simulink model "Linearization2"  (R2022a)
settings: Solver=VariableStepAuto  StartTime=0.0  StopTime=10.0  RelTol=1e-3
undefined symbols (not defined in the file): Aactuator, ac, AeroCoeff, ControlAllocation, DUmax, DUmin, EngineTable, F, fcs, ft, g, hground, IC, kg, LandingGear, Light, LPmethod, m, MIL, Mode_deflection_aileron, Mode_deflection_elevator, Mode_deflection_rudder, Mode_deflection_TVC_y, Mode_deflection_TVC_z, N, Ninv_2nozzle, Ninv_no_nozzle, PIController, s, Sensor, slug, state0, sysID_DAQ, sysID_OBES, Umax_2nozzle, Umax_no_nozzle, Umin_2nozzle, Umin_no_nozzle, WMM2020
libraries: aerolibconvert2 x19, slpidlib x6, simulink x6, sharedutil x4, aerolibatmos2 x3, aerolibwind2 x3, aerolibbdyn x3, aerolibgravity2 x2, sharedtransform x1
(part 4 of 9)

== system Linearization2/F-16 Vehicle Systems Model/sysID_Onboard_Excitation_System/signal generator8 ==
  note: ROM記憶體的指標(Pointer)
  note: 唯讀記憶體，裡面存放波形
  isTurnOn : Inport
  Enable : Inport  Port=2
  sysID_isDone : Inport  Port=3
  Constant1 : Constant  Value=sysID_OBES.rudder.amplitude
  Index Vector : MultiPortSwitch  Inputs=1  SaturateOnIntegerOverflow=off  InputSameDT=off
  Logical Operator1 : Logic  AllPortsSameDT=off  OutDataTypeStr=boolean
  Logical Operator3 : Logic  Operator=NOT  AllPortsSameDT=off  OutDataTypeStr=boolean
  Logical Operator4 : Logic  AllPortsSameDT=off  OutDataTypeStr=boolean
  Pause Counter : Subsystem  TreatAsAtomicUnit=on
  Product : Product
  ROM : Constant  Value=sysID_OBES.rudder.wave
  rudder_delay : Delay  DelayLength=sysID_OBES.rudder.delay/sysID_OBES.Ts  SampleTime=sysID_OBES.Ts
  signal : Outport  OutputWhenDisabled=reset  InitialOutput=0
  isDone : Outport  Port=2
  wires:
  ROM/1 -> Index Vector/2
  Pause Counter/1(CountValue) -> Index Vector/1  "Pointer"
  Pause Counter/2(isCountDone) -> isDone/1
  Constant1/1 -> Product/1
  Index Vector/1 -> Product/2
  Product/1 -> signal/1
  Logical Operator3/1 -> Logical Operator4/2
  sysID_isDone/1 -> Logical Operator3/1  "isDone"
  rudder_delay/1 -> Logical Operator4/1
  Enable/1 -> rudder_delay/1  "isEnable"
  isTurnOn/1 -> Logical Operator1/1  "isTurnOn"
  Logical Operator4/1 -> Logical Operator1/2  "enableSignal"
  Logical Operator1/1 -> Pause Counter/Enable

== system Linearization2/F-16 Vehicle Systems Model/μαβ NDI Controller/command matrix ==
  note: $g_2 {\left(x\right)}={\left[\begin{array}{ccc} g_{\mu_p } & g_{\mu_q } & g_{\mu_r } \\ g_{\alpha_p } & g_{\alpha_q } & g_{\alpha_r } \\ g_{\beta_p } & g_{\beta_q } & g_{\beta_r } \end{array}\right]}={\left[\begin{array}{ccc} \mathrm{cos}\alpha \mathrm{sec}\beta & 0 & \mathrm{sin}\alpha \mathrm{sec}\beta \\ -\mathrm{cos}\alpha \mathrm{tan}\beta & 1 & -\mathrm{sin}\alpha \mathrm{tan}\beta \\ \mathrm{sin}\alpha & 0 & -\mathrm{cos}\alpha \end{array}\right]}$
  α : Inport
  β : Inport  Port=2
  (1,1) : Fcn  Expr=1/cos(u(2)) * cos(u(1))
  (1,2) : Constant  Value=0
  (1,3) : Fcn  Expr=1/cos(u(2)) * sin(u(1))
  (2,1) : Fcn  Expr=-tan(u(2)) * cos(u(1))
  (2,2) : Constant
  (2,3) : Fcn  Expr=-tan(u(2)) * sin(u(1))
  (3,1) : Fcn  Expr=sin(u(1))
  (3,2) : Constant  Value=0
  (3,3) : Fcn  Expr=-cos(u(1))
  Create 3x3 Matrix : sharedutil/Create 3x3 Matrix  aMode=aMode
      settings: SourceProductBaseCode=AE,PW,DR,MT,VE
  Mux4 : Mux  Inputs=2
  g2 : Outport  VectorParamsAs1DForOutWhenUnconnected=off
  wires:
  α/1 -> Mux4/1
  β/1 -> Mux4/2
  Mux4/1 -> (3,3)/1, (3,1)/1, (2,3)/1, (1,1)/1, (1,3)/1, (2,1)/1
  Create 3x3 Matrix/1 -> g2/1
  (2,2)/1 -> Create 3x3 Matrix/5
  (2,1)/1 -> Create 3x3 Matrix/4
  (2,3)/1 -> Create 3x3 Matrix/6
  (1,3)/1 -> Create 3x3 Matrix/3
  (3,1)/1 -> Create 3x3 Matrix/7
  (1,2)/1 -> Create 3x3 Matrix/2
  (3,2)/1 -> Create 3x3 Matrix/8
  (1,1)/1 -> Create 3x3 Matrix/1
  (3,3)/1 -> Create 3x3 Matrix/9

== system Linearization2/F-16 Vehicle Systems Model/μαβ NDI Controller/f2 ==
  note: 有指定port dimensions=3。
      | 否則，雖然可以正常執行程式，
      | 但是t=0會跳出錯誤訊息說下一模塊"attitude NDI"內的矩陣運算的dimensions不一致
  note: mu alpha beta
  note: 11 gravity
  note: 10 T
  note: 9 mass
  note: 8 L
  note: 7 Y
  note: 6 D
  note: 1 Vt alpha beta mu gamma
  note: 11 gravity
  note: 9 mass
  note: 6 Xbar Ybar Zbar
  note: 1 Vinf alpha beta mu gamma
  note: 10 T
  note: 12 f 0 N
  note: 12 f 0 N
  note: 15 chi
  note: 15 chi
  aero V : Inport
  X,Y,Z : Inport  Port=2
  gravity : Inport  Port=3
  Thrust : Inport  Port=4
  LGxyz : Inport  Port=5
  chi : Inport  Port=6
  Add : Sum  Inputs=++++
  Add1 : Sum
  Add2 : Sum
  Drag : Fcn  Expr=-u(6)*cos(u(2))*cos(u(3))-u(7)*sin( u(3) )-u(8)*sin(u(2))*cos(u(3))
  Lift : Fcn  Expr=u(6)*sin(u(2))-u(8)*cos(u(2))
  Mux : Mux  Inputs=3
  Mux1 : Mux  Inputs=9
  Mux2 : Mux  Inputs=2
  Side Force : Fcn  Expr=-u(6)*cos(u(2))*sin(u(3))+u(7)*cos( u(3) )-u(8)*sin(u(2))*sin(u(3))
  f_alpha1 : Fcn  Expr=( -u(8)+u(9)*u(11)*cos(u(5))*cos(u(4))-u(10)*sin(u(2)) ) / ( u(9)*u(1)*cos(u(3)) )
  f_alpha2 : Fcn  Expr=( u(14)*cos(u(5))*cos(u(4))+u(12)*sin(u(15))*sin(u(4))+u(12)*cos(u(15))*cos(u(4))*sin(u(5)) ) / ( u(9)*u(1)*cos(u(3)) )
  f_beta1 : Fcn  Expr=( u(7)*cos(u(3))+u(9)*u(11)*cos(u(5))*sin(u(4))-u(10)*cos(u(2))*sin(u(3)) ) / ( u(9)*u(1) )
  f_beta2 : Fcn  Expr=( u(14)*cos(u(5))*sin(u(4))-u(12)*( cos(u(4))*sin(u(15))-cos(u(15))*sin(u(5))*sin(u(4)) ) / ( u(9)*u(1) ) )
  f_mu1 : Fcn  Expr=u(8)*( tan(u(5))*sin(u(4))+tan(u(3)) ) / ( u(9)*u(1) )
  f_mu2 : Fcn  Expr=(u(7)*tan(u(5))*cos(u(4))*cos(u(3)) -u(9)*u(11)*cos(u(5))*cos(u(4))*tan(u(3)) ) / ( u(9)*u(1) )
  f_mu3 : Fcn  Expr=u(10)*( sin(u(2))*tan(u(5))*sin(u(4)) + sin(u(2))*tan(u(3)) - cos(u(2))*tan(u(5))*cos(u(4))*sin(u(3)) ) / ( u(9)*u(1) )
  f_mu4 : Fcn  Expr="( -u(14)*cos(u(5))*cos(u(4))*tan(u(3))-u(12)*( cos(u(4))*cos(u(15))*sin(u(5))*tan(u(3))+sin(u(15))*tan(u(3))*sin(u(4)) )  ) / ( u(9)*u(1) )"
  m(slugs) : Constant  Value=ac.m
  f2 : Outport  PortDimensions=3  VectorParamsAs1DForOutWhenUnconnected=off
  D : Outport  Port=2  VectorParamsAs1DForOutWhenUnconnected=off
  Y : Outport  Port=3  VectorParamsAs1DForOutWhenUnconnected=off
  L : Outport  Port=4  VectorParamsAs1DForOutWhenUnconnected=off
  wires:
  Mux/1 -> f2/1
  aero V/1 -> Mux1/1, Mux2/1  "Vt, α, β, μ, γ"
  X,Y,Z/1 -> Mux2/2  "Xbar, Ybar, Zbar"
  Mux2/1 -> Lift/1, Drag/1, Side Force/1
  Mux1/1 -> f_beta2/1, f_beta1/1, f_alpha2/1, f_alpha1/1, f_mu4/1, f_mu1/1, f_mu2/1, f_mu3/1
  Drag/1 -> Mux1/2, D/1  "D"
  Side Force/1 -> Mux1/3, Y/1  "Y"
  Lift/1 -> Mux1/4, L/1  "L"
  m(slugs)/1 -> Mux1/5
  Thrust/1 -> Mux1/6  "T"
  gravity/1 -> Mux1/7  "g"
  f_mu2/1 -> Add/2
  f_mu1/1 -> Add/1
  Add/1 -> Mux/1
  f_mu3/1 -> Add/3
  LGxyz/1 -> Mux1/8
  chi/1 -> Mux1/9
  f_alpha1/1 -> Add1/1
  f_alpha2/1 -> Add1/2
  Add1/1 -> Mux/2
  Add2/1 -> Mux/3
  f_beta1/1 -> Add2/1
  f_beta2/1 -> Add2/2
  f_mu4/1 -> Add/4

== system Linearization2/F-16 Vehicle Systems Model/Aerodynamic1/NDI Aerofynamic Coefficients/CXT ==
  note: $C_{X_{\delta_{ra} } } =C_{X_{\delta la} } =\frac{{\hat{X} }_{\delta_e } }{2}∙0.4$
  note: ${\hat{X} }_{\delta_e } =\frac{C_X {\left(\alpha ,\beta ,\delta_e +0.1\right)}-C_X {\left(\alpha ,\beta ,\delta_e -0.1\right)}}{0.2}$
  note: $\delta_e =\frac{\delta_{re} +\delta_{le} }{2}$
  note: 氣動力表格僅提供到攻角到
      | 45度，超過45度後皆採用45
      | 度的氣動力係數
  note: $\Delta C_{X_{LEF} } =C_{X_{LEF} } {\left(\alpha ,\beta \right)}-C_X {\left(\alpha ,\beta ,\delta_e =0°\right)}$
  note: $C_{X,T} =C_X {\left(\alpha ,\beta ,\delta_e \right)}+\Delta C_{X_{LEF} } ∙{\left(1-\frac{\delta_{LEF} }{25°}\right)}+\frac{q\overset{-}{c} }{2V_T }∙{\left[C_{X_q } {\left(\alpha \right)}+\Delta C_{X_{q_{LEF} } } {\left(\alpha \right)}∙{\left(1-\frac{\delta_{LEF} }{25°}\right)}\right]}+\mathrm{\ }\Delta C_{X_{SB} } {\left(\alpha \right)}∙{\left(\frac{\delta_{SB} }{60°}\right)}+C_{X_{\delta_{ra} } } {∙\delta }_{ra} +C_{X_{\delta_{la} } } {∙\delta }_{la}$
  note: 體軸 x 方向之氣動力係數 (total x-axis force coefficient)：
  note: ${\left(1-\frac{\delta_{LEF} }{25°}\right)}$
  note: $C_{X_{\delta_{ra} } } =C_{X_{\delta la} } =\frac{{\hat{X} }_{\delta_e } }{2}∙0.4$
  note: ${\hat{X} }_{\delta_e } =\frac{C_X {\left(\alpha ,\beta ,\delta_e +0.1\right)}-C_X {\left(\alpha ,\beta ,\delta_e -0.1\right)}}{0.2}$
  alpha (deg) : Inport
  beta (deg) : Inport  Port=2
  right elevator (deg) : Inport  Port=3
  left elevator (deg) : Inport  Port=4
  dlef : Inport  Port=5
  qc_2v : Inport  Port=6
  sb : Inport  Port=7
  right aileron : Inport  Port=8
  left aileron : Inport  Port=9
  Add : Sum  Inputs=+-
  Add1 : Sum  Inputs=+++++
  Add{2..4,7} (4 alike) : Sum
  Add5 : Sum  Inputs=+-
  Add6 : Sum  Inputs=+-
  Constant : Constant  Value=0.1
  Constant1 : Constant  Value=0.1
  Constant2 : Constant  Value=0.2
  Cx : Interpolation_n-D  NumberOfTableDimensions=3  Table=AeroCoeff.Cx
      settings: InputPortMap=u0,u1,u2,u3,u4,u5
  Cx1 : Interpolation_n-D  NumberOfTableDimensions=3  Table=AeroCoeff.Cx
      settings: InputPortMap=u0,u1,u2,u3,u4,u5
  Cx2 : Interpolation_n-D  NumberOfTableDimensions=3  Table=AeroCoeff.Cx
      settings: InputPortMap=u0,u1,u2,u3,u4,u5
  Cx_elevator0 : Interpolation_n-D  Table=AeroCoeff.Cx_elevator0
  Cx_lef : Interpolation_n-D  Table=AeroCoeff.Cx_lef
  Cx_q : Interpolation_n-D  NumberOfTableDimensions=1  Table=AeroCoeff.Cx_q
      settings: InputPortMap=u0,u1
  Cx_q_lef : Interpolation_n-D  NumberOfTableDimensions=1  Table=AeroCoeff.Cx_q_lef
      settings: InputPortMap=u0,u1
  Divide : Product  Inputs=*/
  Gain : Gain  Gain=20
  Gain1 : Gain  Gain=(1/2)*0.4
  Gain3 : Gain  Gain=20
  Gain4 : Gain  Gain=1/2
  Product{,1..5} (6 alike) : Product
  alpha Prelookup : PreLookup  BreakpointsData=AeroCoeff.alpha_prelookup  IndexSearchMethod=Linear search  BeginIndexSearchUsingPreviousIndexResult=on  DiagnosticForOutOfRangeInput=Warning
  beta Prelookup : PreLookup  BreakpointsData=AeroCoeff.beta_prelookup  IndexSearchMethod=Linear search  BeginIndexSearchUsingPreviousIndexResult=on  DiagnosticForOutOfRangeInput=Warning
  dCX_sb : Interpolation_n-D  NumberOfTableDimensions=1  Table=AeroCoeff.dCX_sb
      settings: InputPortMap=u0,u1
  elevator Prelookup : PreLookup  BreakpointsData=AeroCoeff.elevator_prelookup2  IndexSearchMethod=Linear search  BeginIndexSearchUsingPreviousIndexResult=on  DiagnosticForOutOfRangeInput=Warning
  elevator Prelookup1 : PreLookup  BreakpointsData=AeroCoeff.elevator_prelookup2  IndexSearchMethod=Linear search  BeginIndexSearchUsingPreviousIndexResult=on  DiagnosticForOutOfRangeInput=Warning
  elevator Prelookup2 : PreLookup  BreakpointsData=AeroCoeff.elevator_prelookup2  IndexSearchMethod=Linear search  BeginIndexSearchUsingPreviousIndexResult=on  DiagnosticForOutOfRangeInput=Warning
  Cx_tot : Outport  VectorParamsAs1DForOutWhenUnconnected=off
  wires:
  beta Prelookup/2 -> Cx2/4, Cx1/4, Cx_elevator0/4, Cx_lef/4, Cx/4
  alpha (deg)/1 -> alpha Prelookup/1
  beta Prelookup/1 -> Cx2/3, Cx1/3, Cx_elevator0/3, Cx_lef/3, Cx/3
  Cx_lef/1 -> Add/1
  alpha Prelookup/1 -> Cx2/1, Cx1/1, dCX_sb/1, Cx_q_lef/1, Cx_q/1, Cx_elevator0/1, Cx/1, Cx_lef/1
  elevator Prelookup/2 -> Cx/6
  Add3/1 -> Gain4/1
  beta (deg)/1 -> beta Prelookup/1
  Add/1 -> Product/1
  alpha Prelookup/2 -> Cx1/2, Cx2/2, dCX_sb/2, Cx_q_lef/2, Cx_q/2, Cx_elevator0/2, Cx_lef/2, Cx/2
  Product/1 -> Add1/2
  elevator Prelookup/1 -> Cx/5
  Add2/1 -> Product2/1
  Cx/1 -> Add1/1
  Cx_elevator0/1 -> Add/2
  Cx_q_lef/1 -> Product1/1
  Product1/1 -> Add2/2
  Cx_q/1 -> Add2/1
  dlef/1 -> Product/2, Product1/2
  Product2/1 -> Add1/3
  Add1/1 -> Cx_tot/1
  qc_2v/1 -> Product2/2
  dCX_sb/1 -> Product3/1
  sb/1 -> Product3/2
  Product3/1 -> Add1/4
  right elevator (deg)/1 -> Add3/1
  left elevator (deg)/1 -> Add3/2
  Cx2/1 -> Add6/2
  Divide/1 -> Gain1/1
  Constant/1 -> Add4/2
  Add5/1 -> elevator Prelookup2/1
  Product5/1 -> Add7/2
  Gain1/1 -> Product5/1, Product4/1
  Add6/1 -> Divide/1
  Constant1/1 -> Add5/2
  Constant2/1 -> Divide/2
  Cx1/1 -> Add6/1
  Product4/1 -> Add7/1
  Add4/1 -> elevator Prelookup1/1
  elevator Prelookup1/1 -> Cx1/5
  elevator Prelookup1/2 -> Cx1/6
  elevator Prelookup2/1 -> Cx2/5
  elevator Prelookup2/2 -> Cx2/6
  right aileron/1 -> Gain/1
  left aileron/1 -> Gain3/1
  Gain/1 -> Product4/2
  Gain3/1 -> Product5/2
  Add7/1 -> Add1/5
  Gain4/1 -> elevator Prelookup/1, Add4/1, Add5/1

== system Linearization2/F-16 Vehicle Systems Model/Aerodynamic1/NDI Aerofynamic Coefficients/CYT ==
  note: ${\left[\Delta C_{Y_{\delta_a } } +\Delta C_{Y_{{\delta_a }_{LEF} } } ∙{\left(1-\frac{\delta_{LEF} }{25°}\right)}\right]}$
  note: $\Delta C_{Y_{\delta_r } }$
  note: $\Delta C_{Y_{{\delta_a }_{LEF} } } =C_{Y_{{\delta_a =20°}_{LEF} } } {\left(\alpha ,\beta \right)}-C_{Y_{LEF} } {\left(\alpha ,\beta \right)}-\Delta C_{Y_{\delta_a } }$
  note: $\Delta C_{Y_{\delta_a } } =C_{Y_{\delta_a =20°} } {\left(\alpha ,\beta \right)}-C_Y {\left(\alpha ,\beta \right)}$
  note: ${\left(1-\frac{\delta_{LEF} }{25°}\right)}$
  note: $\frac{{\left[\Delta C_{Y_{\delta_a } } +\Delta C_{Y_{{\delta_a }_{LEF} } } ∙{\left(1-\frac{\delta_{LEF} }{25°}\right)}\right]}}{2}$
  note: 氣動力表格僅提供到攻角到
      | 45度，超過45度後皆採用45
      | 度的氣動力係數
  note: 氣動力表格僅提供到攻角到
      | 45度，超過45度後皆採用45
      | 度的氣動力係數
  note: 體軸 y 方向之氣動力係數 (total y-axis force coefficient)：
  note: $\Delta C_{Y_{LEF} }=C_{Y_{LEF} } {\left(\alpha ,\beta \right)}\ \ -C_Y {\left(\alpha ,\beta \right)}$
  note: $\Delta C_{Y_{\delta_r } }=C_{Y_{\delta_r =30°} } {\left(\alpha ,\beta \right)}-C_Y {\left(\alpha ,\beta \right)}$
  note: $C_{Y,T} \ \ \ =\ \ \ \ C_Y {\left(\alpha ,\beta \right)}+\Delta C_{Y_{LEF} } ∙{\left(1-\frac{\delta_{LEF} }{25°}\right)}+\frac{pb}{2V_T }∙{\left[C_{Y_p } {\left(\alpha \right)}+\Delta C_{{Y_p }_{LEF} } {\left(\alpha \right)}∙{\left(1-\frac{\delta_{LEF} }{25°}\right)}\right]}+\ \frac{rb}{2V_T }∙{\left[C_{Y_r } {\left(\alpha \right)}+\Delta C_{{Y_r }_{LEF} } {\left(\alpha \right)}∙{\left(1-\frac{\delta_{LEF} }{25°}\right)}\right]}+\Delta C_{Y_{\delta_r } } ∙{\left(\frac{\delta_r }{30°}\right)}+\frac{{\left[\Delta C_{Y_{\delta_a } } +\Delta C_{Y_{{\delta_a }_{LEF} } } ∙{\left(1-\frac{\delta_{LEF} }{25°}\right)}\right]}}{2}∙{\left(\frac{\delta_{ra} }{20°}\right)}-\frac{{\left[\Delta C_{Y_{\delta_a } } +\Delta C_{Y_{{\delta_a }_{LEF} } } ∙{\left(1-\frac{\delta_{LEF} }{25°}\right)}\right]}}{2}∙{\left(\frac{\delta_{la} }{20°}\right)}{+C}_{Y_{\delta_{re} } } ∙{\left(\frac{\delta_{re} }{25°}\right)}-C_{Y_{\delta_{le} } } ∙{\left(\frac{\delta_{le} }{25°}\right)}$
  note: $\Delta C_{Y_{{\delta_a }_{LEF} } } =C_{Y_{{\delta_a =20°}_{LEF} } } {\left(\alpha ,\beta \right)}-C_{Y_{LEF} } {\left(\alpha ,\beta \right)}-\Delta C_{Y_{\delta_a } }$
  note: $\Delta C_{Y_{\delta_a } }=C_{Y_{\delta_a =20°} } {\left(\alpha ,\beta \right)}-C_Y {\left(\alpha ,\beta \right)}$
  note: $\Delta C_{Y_{\delta_r } } =C_{Y_{\delta_r =30°} } {\left(\alpha ,\beta \right)}-C_Y {\left(\alpha ,\beta \right)}$
  note: $C_{Y_{\delta_{re} } } =C_{Y_{\delta_{le} } } =\frac{\Delta C_{Y_{\delta_a } } }{2}∙0.68$
  note: $C_{Y_{\delta_{re} } } =C_{Y_{\delta_{le} } } =\frac{\Delta C_{Y_{\delta_a } } }{2}∙0.68$
  alpha (deg) : Inport
  beta (deg) : Inport  Port=2
  dlef : Inport  Port=3
  right aileron : Inport  Port=4
  left aileron : Inport  Port=5
  drud : Inport  Port=6
  rb_2v : Inport  Port=7
  pb_2v : Inport  Port=8
  Add : Sum  Inputs=-+
  Add1 : Sum  Inputs=-+
  Add2 : Sum  Inputs=+--
  Add3 : Sum  Inputs=+-
  Add4 : Sum  Inputs=++++++
  Add5 : Sum
  Add6 : Sum
  Add7 : Sum
  Add8 : Sum  Inputs=++++
  Add9 : Sum  Inputs=+-
  CY : Interpolation_n-D  Table=AeroCoeff.CY
  CY_delta_ail : Interpolation_n-D  Table=AeroCoeff.CY_delta_ail
  CY_delta_ail_lef : Interpolation_n-D  Table=AeroCoeff.CY_delta_ail_lef
  CY_delta_r : Interpolation_n-D  Table=AeroCoeff.CY_delta_r
  CY_lef : Interpolation_n-D  Table=AeroCoeff.CY_lef
  CY_p : Interpolation_n-D  NumberOfTableDimensions=1  Table=AeroCoeff.CY_p
      settings: InputPortMap=u0,u1
  CY_r : Interpolation_n-D  NumberOfTableDimensions=1  Table=AeroCoeff.CY_r
      settings: InputPortMap=u0,u1
  Gain : Gain  Gain=0.5
  Gain1 : Gain  Gain=1/2
  Gain2 : Gain  Gain=(1/2)*0.68
  Product{,1..7} (8 alike) : Product
  alpha Prelookup : PreLookup  BreakpointsData=AeroCoeff.alpha_prelookup  IndexSearchMethod=Linear search  BeginIndexSearchUsingPreviousIndexResult=on  DiagnosticForOutOfRangeInput=Warning
  beta Prelookup : PreLookup  BreakpointsData=AeroCoeff.beta_prelookup  IndexSearchMethod=Linear search  BeginIndexSearchUsingPreviousIndexResult=on  DiagnosticForOutOfRangeInput=Warning
  dCY_p_lef : Interpolation_n-D  NumberOfTableDimensions=1  Table=AeroCoeff.dCY_p_lef
      settings: InputPortMap=u0,u1
  dCY_r_lef : Interpolation_n-D  NumberOfTableDimensions=1  Table=AeroCoeff.dCY_r_lef
      settings: InputPortMap=u0,u1
  Cy_tot : Outport  VectorParamsAs1DForOutWhenUnconnected=off
  Cy_tot_n_mom : Outport  Port=2  VectorParamsAs1DForOutWhenUnconnected=off
  Cy_tot_n_da : Outport  Port=3  VectorParamsAs1DForOutWhenUnconnected=off
  Cy_tot_n_dr : Outport  Port=4  VectorParamsAs1DForOutWhenUnconnected=off
  Cy_tot_n_de : Outport  Port=5  VectorParamsAs1DForOutWhenUnconnected=off
  wires:
  Add3/1 -> Cy_tot_n_dr/1, Product3/1
  beta Prelookup/2 -> CY_delta_r/4, CY_delta_ail_lef/4, CY_delta_ail/4, CY/4, CY_lef/4
  beta Prelookup/1 -> CY_delta_r/3, CY_delta_ail_lef/3, CY_delta_ail/3, CY/3, CY_lef/3
  Product7/1 -> Add4/6, Add8/4
  dlef/1 -> Product1/2, Product/2, Product4/2, Product6/1
  alpha Prelookup/1 -> dCY_p_lef/1, CY_p/1, dCY_r_lef/1, CY_r/1, CY_delta_r/1, CY_delta_ail_lef/1, CY_delta_ail/1, CY_lef/1, CY/1
  Add4/1 -> Cy_tot/1
  Add5/1 -> Gain1/1, Product2/1
  CY_p/1 -> Add7/1
  CY_lef/1 -> Add/2, Add2/2
  Add/1 -> Product/1
  dCY_p_lef/1 -> Product6/2
  CY_delta_r/1 -> Add3/1
  CY_delta_ail_lef/1 -> Add2/1
  dCY_r_lef/1 -> Product4/1
  alpha (deg)/1 -> alpha Prelookup/1
  CY_r/1 -> Add6/1
  Product4/1 -> Add6/2
  Add2/1 -> Product1/1
  Product3/1 -> Add4/4
  CY/1 -> Add8/1, Add4/1, Add/1, Add1/1, Add3/2
  Product2/1 -> Add4/3
  Product/1 -> Add4/2, Add8/2
  alpha Prelookup/2 -> CY_p/2, dCY_p_lef/2, dCY_r_lef/2, CY_r/2, CY_delta_r/2, CY_delta_ail_lef/2, CY_delta_ail/2, CY_lef/2, CY/2
  Product6/1 -> Add7/2
  Add6/1 -> Product5/2
  Add7/1 -> Product7/2
  Product5/1 -> Add4/5, Add8/3
  Product1/1 -> Add5/2
  CY_delta_ail/1 -> Add1/2
  beta (deg)/1 -> beta Prelookup/1
  drud/1 -> Product3/2
  pb_2v/1 -> Product7/1
  rb_2v/1 -> Product5/1
  Add8/1 -> Cy_tot_n_mom/1
  right aileron/1 -> Add9/1
  left aileron/1 -> Add9/2
  Add9/1 -> Gain/1
  Gain2/1 -> Cy_tot_n_de/1
  Gain/1 -> Product2/2
  Gain1/1 -> Cy_tot_n_da/1
  Add1/1 -> Gain2/1, Add2/3, Add5/1

== system Linearization2/F-16 Vehicle Systems Model/Aerodynamic1/NDI Aerofynamic Coefficients/CZT ==
  note: ${\hat{Z} }_{\delta_e } =\frac{C_Z {\left(\alpha ,\beta ,\delta_e +0.1\right)}-C_Z {\left(\alpha ,\beta ,\delta_e -0.1\right)}}{0.2}$
  note: ${\hat{Z} }_{\delta_e }$
  note: CZ
  note: 氣動力表格僅提供到攻角到
      | 45度，超過45度後皆採用45
      | 度的氣動力係數
  note: $\Delta C_{Z_{LEF} } =C_{Z_{LEF} } {\left(\alpha ,\beta \right)}-C_Z {\left(\alpha ,\beta ,\delta_e =0°\right)}$
  note: $C_{Z,T} =C_Z {\left(\alpha ,\beta ,\delta_e \right)}+\Delta C_{Z_{LEF} } ∙{\left(1-\frac{\delta_{LEF} }{25°}\right)}+\frac{q\overset{-}{c} }{2V_T }∙{\left[C_{Z_q } {\left(\alpha \right)}+\Delta C_{Z_{q_{LEF} } } {\left(\alpha \right)}∙{\left(1-\frac{\delta_{LEF} }{25°}\right)}\right]}+\ \Delta C_{Z_{SB} } {\left(\alpha \right)}∙{\left(\frac{\delta_{SB} }{60°}\right)}+C_{Z_{\delta ra} } \delta_{ra} +C_{Z_{\delta la} } \delta_{la}$
  note: 體軸 z 方向之氣動力係數 (total z-axis force coefficient)：
  note: ${\left(1-\frac{\delta_{LEF} }{25°}\right)}$
  note: $C_{Z_{\delta ra} } =C_{Z_{\delta la} } =\frac{{\hat{Z} }_{\delta_e } }{2}∙0.4$
  note: $\delta_e =\frac{\delta_{re} +\delta_{le} }{2}$
  note: $\hat{Z} =\bar{q} S\bar{C} {\left\{C_{Z,T} -{\hat{Z} }_{\delta_e } ∙\delta_e \right\}}$
  note: 註： $\bar{q} S\bar{C}$ 在模塊外面乘
  note: ${\hat{Z} }_{\delta_e } =\frac{C_Z {\left(\alpha ,\beta ,\delta_e +0.1\right)}-C_Z {\left(\alpha ,\beta ,\delta_e -0.1\right)}}{0.2}$
  note: $C_{Z_{\delta ra} } =C_{Z_{\delta la} } =\frac{{\hat{Z} }_{\delta_e } }{2}∙0.4$
  alpha (deg) : Inport
  beta (deg) : Inport  Port=2
  right elevator (deg) : Inport  Port=3
  left elevator (deg) : Inport  Port=4
  dlef : Inport  Port=5
  qc_2v : Inport  Port=6
  sb : Inport  Port=7
  Add : Sum  Inputs=+-
  Add1 : Sum  Inputs=++++
  Add2 : Sum
  Add3 : Sum
  Add4 : Sum  Inputs=+-
  Add5 : Sum  Inputs=+-
  Bias : Bias  Bias=0.1  SaturateOnIntegerOverflow=off
  Bias1 : Bias  Bias=-0.1  SaturateOnIntegerOverflow=off
  CZ : Interpolation_n-D  NumberOfTableDimensions=3  Table=AeroCoeff.CZ
      settings: InputPortMap=u0,u1,u2,u3,u4,u5
  CZ_elevator0 : Interpolation_n-D  Table=AeroCoeff.CZ_elevator0
  CZ_lef : Interpolation_n-D  Table=AeroCoeff.CZ_lef
  CZ_q : Interpolation_n-D  NumberOfTableDimensions=1  Table=AeroCoeff.CZ_q
      settings: InputPortMap=u0,u1
  Constant : Constant  Value=0.2
  Divide : Product  Inputs=*/
  Gain1 : Gain  Gain=(1/2)*0.4
  Gain4 : Gain  Gain=1/2
  Product{,1..4} (5 alike) : Product
  alpha Prelookup : PreLookup  BreakpointsData=AeroCoeff.alpha_prelookup  IndexSearchMethod=Linear search  BeginIndexSearchUsingPreviousIndexResult=on  DiagnosticForOutOfRangeInput=Warning
  beta Prelookup : PreLookup  BreakpointsData=AeroCoeff.beta_prelookup  IndexSearchMethod=Linear search  BeginIndexSearchUsingPreviousIndexResult=on  DiagnosticForOutOfRangeInput=Warning
  dCZ_q_lef : Interpolation_n-D  NumberOfTableDimensions=1  Table=AeroCoeff.dCZ_q_lef
      settings: InputPortMap=u0,u1
  dCZ_sb : Interpolation_n-D  NumberOfTableDimensions=1  Table=AeroCoeff.dCZ_sb
      settings: InputPortMap=u0,u1
  elevator Prelookup : PreLookup  BreakpointsData=AeroCoeff.elevator_prelookup2  IndexSearchMethod=Linear search  BeginIndexSearchUsingPreviousIndexResult=on  DiagnosticForOutOfRangeInput=Warning
  elevator Prelookup1 : PreLookup  BreakpointsData=AeroCoeff.elevator_prelookup2  IndexSearchMethod=Linear search  BeginIndexSearchUsingPreviousIndexResult=on  DiagnosticForOutOfRangeInput=Warning
  elevator Prelookup2 : PreLookup  BreakpointsData=AeroCoeff.elevator_prelookup2  IndexSearchMethod=Linear search  BeginIndexSearchUsingPreviousIndexResult=on  DiagnosticForOutOfRangeInput=Warning
  same as CZ : Interpolation_n-D  NumberOfTableDimensions=3  Table=AeroCoeff.CZ
      settings: InputPortMap=u0,u1,u2,u3,u4,u5
  same_as_CZ : Interpolation_n-D  NumberOfTableDimensions=3  Table=AeroCoeff.CZ
      settings: InputPortMap=u0,u1,u2,u3,u4,u5
  Cz_tot_plus : Outport  VectorParamsAs1DForOutWhenUnconnected=off
  Cz_tot_minus : Outport  Port=2  VectorParamsAs1DForOutWhenUnconnected=off
  Cz_tot_m_de : Outport  Port=3  VectorParamsAs1DForOutWhenUnconnected=off
  Cz_tot_m_da : Outport  Port=4  VectorParamsAs1DForOutWhenUnconnected=off
  Cz_tot : Outport  Port=5  VectorParamsAs1DForOutWhenUnconnected=off
  Cz_tot_hat : Outport  Port=6  VectorParamsAs1DForOutWhenUnconnected=off
  wires:
  Product2/1 -> Add1/3
  alpha Prelookup/2 -> same as CZ/2, same_as_CZ/2, dCZ_sb/2, dCZ_q_lef/2, CZ_q/2, CZ_elevator0/2, CZ_lef/2, CZ/2
  elevator Prelookup/1 -> CZ/5
  CZ_q/1 -> Add2/1
  beta Prelookup/2 -> same as CZ/4, same_as_CZ/4, CZ_elevator0/4, CZ/4, CZ_lef/4
  CZ_lef/1 -> Add/1
  dCZ_q_lef/1 -> Product1/1
  Product1/1 -> Add2/2
  Add2/1 -> Product2/1
  CZ_elevator0/1 -> Add/2
  Add/1 -> Product/1
  dlef/1 -> Product1/2, Product/2
  Product/1 -> Add1/2
  CZ/1 -> Add1/1
  beta Prelookup/1 -> same as CZ/3, same_as_CZ/3, CZ_elevator0/3, CZ_lef/3, CZ/3
  alpha Prelookup/1 -> same as CZ/1, same_as_CZ/1, dCZ_sb/1, dCZ_q_lef/1, CZ_q/1, CZ_elevator0/1, CZ_lef/1, CZ/1
  alpha (deg)/1 -> alpha Prelookup/1
  elevator Prelookup/2 -> CZ/6
  qc_2v/1 -> Product2/2
  beta (deg)/1 -> beta Prelookup/1
  right elevator (deg)/1 -> Add3/1
  Bias/1 -> elevator Prelookup1/1
  Bias1/1 -> elevator Prelookup2/1
  elevator Prelookup1/2 -> same_as_CZ/6
  elevator Prelookup1/1 -> same_as_CZ/5
  elevator Prelookup2/2 -> same as CZ/6
  elevator Prelookup2/1 -> same as CZ/5
  same_as_CZ/1 -> Cz_tot_plus/1, Add4/1
  same as CZ/1 -> Cz_tot_minus/1, Add4/2
  sb/1 -> Product3/2
  dCZ_sb/1 -> Product3/1
  Product3/1 -> Add1/4
  left elevator (deg)/1 -> Add3/2
  Add3/1 -> Gain4/1
  Add4/1 -> Divide/1
  Constant/1 -> Divide/2
  Add1/1 -> Cz_tot/1, Add5/1
  Product4/1 -> Add5/2
  Add5/1 -> Cz_tot_hat/1
  Divide/1 -> Cz_tot_m_de/1, Gain1/1, Product4/2
  Gain1/1 -> Cz_tot_m_da/1
  Gain4/1 -> Bias/1, Bias1/1, Product4/1, elevator Prelookup/1

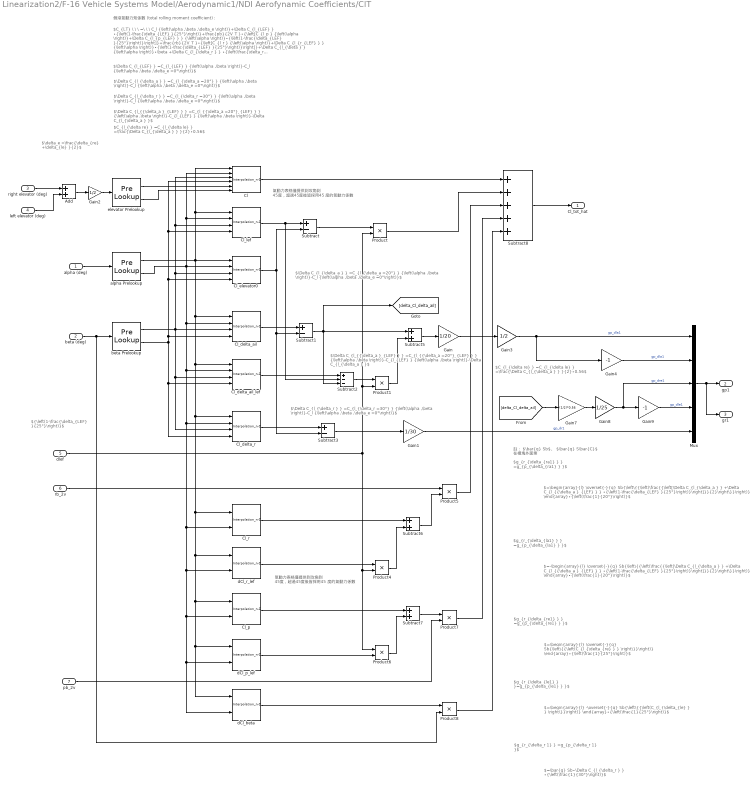
== system Linearization2/F-16 Vehicle Systems Model/Aerodynamic1/NDI Aerofynamic Coefficients/ClT ==
  note: $C_{l_{\delta re} } =C_{l_{\delta le} } =\frac{\Delta C_{l_{\delta_a } } }{2}∙0.56$
  note: 氣動力表格僅提供到攻角到
      | 45度，超過45度後皆採用45
      | 度的氣動力係數
  note: 氣動力表格僅提供到攻角到
      | 45度，超過45度後皆採用45
      | 度的氣動力係數
  note: $\Delta C_{l_{LEF} } =C_{l_{LEF} } {\left(\alpha ,\beta \right)}-C_l {\left(\alpha ,\beta ,\delta_e =0°\right)}$
  note: $\Delta C_{l_{\delta_a } } =C_{l_{\delta_a =20°} } {\left(\alpha ,\beta \right)}-C_l {\left(\alpha ,\beta ,\delta_e =0°\right)}$
  note: $C_{l,T} \ \ \ =\ \ \ C_l {\left(\alpha ,\beta ,\delta_e \right)}+\Delta C_{l_{LEF} } ∙{\left(1-\frac{\delta_{LEF} }{25°}\right)}+\frac{pb}{2V_T }∙{\left[C_{l_p } {\left(\alpha \right)}+\Delta C_{l_{p_{LEF} } } {\left(\alpha \right)}∙{\left(1-\frac{\delta_{LEF} }{25°}\right)}\right]}+\frac{rb}{2V_T }∙{\left[C_{l_r } {\left(\alpha \right)}+\Delta C_{l_{r_{LEF} } } {\left(\alpha \right)}∙{\left(1-\frac{\delta_{LEF} }{25°}\right)}\right]}+\Delta C_{l_{\beta } } {\left(\alpha \right)}∙\beta +\Delta C_{l_{\delta_r } } ∙{\left(\frac{\delta_r }{30°}\right)}+\frac{{\left[\Delta C_{l_{\delta_a } } +\Delta C_{l_{{\delta_a }_{LEF} } } ∙{\left(1-\frac{\delta_{LEF} }{25°}\right)}\right]}}{2}∙{\left(\frac{\delta_{ra} }{20°}\right)}-\frac{{\left[\Delta C_{l_{\delta_a } } +\Delta C_{l_{{\delta_a }_{LEF} } } ∙{\left(1-\frac{\delta_{LEF} }{25°}\right)}\right]}}{2}∙{\left(\frac{\delta_{la} }{20°}\right)}+C_{l_{\delta re} } ∙{\left(\frac{\delta_{re} }{25°}\right)}-C_{l_{\delta le} } ∙{\left(\frac{\delta_{le} }{25°}\right)}$
  note: 側滾氣動力矩係數 (total rolling moment coefficient)：
  note: $\Delta C_{l_{\delta_r } } =C_{l_{\delta_r =30°} } {\left(\alpha ,\beta \right)}-C_l {\left(\alpha ,\beta ,\delta_e =0°\right)}$
  note: $\Delta C_{l_{{\delta_a }_{LEF} } } =C_{l_{{\delta_a =20°}_{LEF} } } {\left(\alpha ,\beta \right)}-C_{l_{LEF} } {\left(\alpha ,\beta \right)}-\Delta C_{l_{\delta_a } }$
  note: ${\left(1-\frac{\delta_{LEF} }{25°}\right)}$
  note: 註： $\bar{q} Sb$ 、 $\bar{q} S\bar{C}$ 在模塊外面乘
  note: $\Delta C_{l_{\delta_r } } =C_{l_{\delta_r =30°} } {\left(\alpha ,\beta \right)}-C_l {\left(\alpha ,\beta ,\delta_e =0°\right)}$
  note: $\Delta C_{l_{{\delta_a }_{LEF} } } =C_{l_{{\delta_a =20°}_{LEF} } } {\left(\alpha ,\beta \right)}-C_{l_{LEF} } {\left(\alpha ,\beta \right)}-\Delta C_{l_{\delta_a } }$
  note: $\Delta C_{l_{\delta_a } } =C_{l_{\delta_a =20°} } {\left(\alpha ,\beta \right)}-C_l {\left(\alpha ,\beta ,\delta_e =0°\right)}$
  note: $\delta_e =\frac{\delta_{re} +\delta_{le} }{2}$
  note: $=\begin{array}{l} \overset{-}{q} Sb{\left\{{\left(\frac{{\left[\Delta C_{l_{\delta_a } } +\Delta C_{l_{{\delta_a }_{LEF} } } ∙{\left(1-\frac{\delta_{LEF} }{25°}\right)}\right]}}{2}\right\}}\right)} \end{array}∙{\left(\frac{1}{20°}\right)}$
  note: $g_{r_{\delta_{ra1} } } =g_{p_{\delta_{ra1} } }$
  note: $g_{r_{\delta_{la1} } } =g_{p_{\delta_{la1} } }$
  note: $=-\begin{array}{l} \overset{-}{q} Sb{\left\{{\left(\frac{{\left[\Delta C_{l_{\delta_a } } +\Delta C_{l_{{\delta_a }_{LEF} } } ∙{\left(1-\frac{\delta_{LEF} }{25°}\right)}\right]}}{2}\right\}}\right)} \end{array}∙{\left(\frac{1}{20°}\right)}$
  note: $g_{r_{\delta_{re1} } } =g_{p_{\delta_{re1} } }$
  note: $=\begin{array}{l} \overset{-}{q} Sb{\left\{{\left(C_{l_{\delta_{re} } } \right\}}\right)} \end{array}∙{\left(\frac{1}{25°}\right)}$
  note: $g_{r_{\delta_{le1} } }=g_{p_{\delta_{le1} } }$
  note: $=\begin{array}{l} -\overset{-}{q} Sb{\left\{{\left(C_{l_{\delta_{le} } } \right\}}\right)} \end{array}∙{\left(\frac{1}{25°}\right)}$
  note: $g_{r_{\delta_r 1} } =g_{p_{\delta_r 1} }$
  note: $=\bar{q} Sb∙\Delta C_{l_{\delta_r } } ∙{\left(\frac{1}{30°}\right)}$
  note: $C_{l_{\delta re} } =C_{l_{\delta le} } =\frac{\Delta C_{l_{\delta_a } } }{2}∙0.56$
  alpha (deg) : Inport
  beta (deg) : Inport  Port=2
  right elevator (deg) : Inport  Port=3
  left elevator (deg) : Inport  Port=4
  dlef : Inport  Port=5
  rb_2v : Inport  Port=6
  pb_2v : Inport  Port=7
  Add : Sum
  Cl : Interpolation_n-D  NumberOfTableDimensions=3  Table=AeroCoeff.Cl
      settings: InputPortMap=u0,u1,u2,u3,u4,u5
  Cl_delta_ail : Interpolation_n-D  Table=AeroCoeff.Cl_delta_ail  InternalRulePriority=Speed
  Cl_delta_ail_lef : Interpolation_n-D  Table=AeroCoeff.Cl_delta_ail_lef  InternalRulePriority=Speed
  Cl_delta_r : Interpolation_n-D  Table=AeroCoeff.Cl_delta_r  InternalRulePriority=Speed
  Cl_elevator0 : Interpolation_n-D  Table=AeroCoeff.Cl_elevator0
  Cl_lef : Interpolation_n-D  Table=AeroCoeff.Cl_lef  InternalRulePriority=Speed
  Cl_p : Interpolation_n-D  NumberOfTableDimensions=1  Table=AeroCoeff.Cl_p  InternalRulePriority=Speed
      settings: InputPortMap=u0,u1
  Cl_r : Interpolation_n-D  NumberOfTableDimensions=1  Table=AeroCoeff.Cl_r  InternalRulePriority=Speed
      settings: InputPortMap=u0,u1
  Gain : Gain  Gain=1/20
  Gain1 : Gain  Gain=1/30
  Gain2 : Gain  Gain=1/2
  Gain3 : Gain  Gain=1/2
  Gain4 : Gain  Gain=-1
  Gain7 : Gain  Gain=(1/2)*0.56
  Gain8 : Gain  Gain=1/25
  Gain9 : Gain  Gain=-1
  Mux : Mux  Inputs=5
  Product{,1,4..8} (7 alike) : Product
  Subtract : Sum  Inputs=+-
  Subtract1 : Sum  Inputs=+-
  Subtract2 : Sum  Inputs=+--
  Subtract3 : Sum  Inputs=+-
  Subtract5 : Sum
  Subtract6 : Sum
  Subtract7 : Sum
  Subtract8 : Sum  Inputs=+++++
  alpha Prelookup : PreLookup  BreakpointsData=AeroCoeff.alpha_prelookup  IndexSearchMethod=Linear search  BeginIndexSearchUsingPreviousIndexResult=on  DiagnosticForOutOfRangeInput=Warning
  beta Prelookup : PreLookup  BreakpointsData=AeroCoeff.beta_prelookup  IndexSearchMethod=Linear search  BeginIndexSearchUsingPreviousIndexResult=on  DiagnosticForOutOfRangeInput=Warning
  dCl_beta : Interpolation_n-D  NumberOfTableDimensions=1  Table=AeroCoeff.dCl_beta  InternalRulePriority=Speed
      settings: InputPortMap=u0,u1
  dCl_p_lef : Interpolation_n-D  NumberOfTableDimensions=1  Table=AeroCoeff.dCl_p_lef  InternalRulePriority=Speed
      settings: InputPortMap=u0,u1
  dCl_r_lef : Interpolation_n-D  NumberOfTableDimensions=1  Table=AeroCoeff.dCl_r_lef  InternalRulePriority=Speed
      settings: InputPortMap=u0,u1
  elevator Prelookup : PreLookup  BreakpointsData=AeroCoeff.elevator_prelookup1  IndexSearchMethod=Linear search  BeginIndexSearchUsingPreviousIndexResult=on  DiagnosticForOutOfRangeInput=Warning
  Cl_tot_hat : Outport  VectorParamsAs1DForOutWhenUnconnected=off
  gp1 : Outport  Port=2
  gr1 : Outport  Port=3
  wires:
  Cl_elevator0/1 -> Subtract3/2, Subtract1/2, Subtract/2
  beta Prelookup/1 -> Cl/3, Cl_lef/3, Cl_elevator0/3, Cl_delta_ail_lef/3, Cl_delta_r/3, Cl_delta_ail/3
  Cl_delta_r/1 -> Subtract3/1
  Cl_lef/1 -> Subtract2/2, Subtract/1
  Subtract/1 -> Product/1
  Product6/1 -> Subtract7/2
  alpha Prelookup/1 -> dCl_r_lef/1, dCl_p_lef/1, dCl_beta/1, Cl_p/1, Cl_r/1, Cl_delta_r/1, Cl_delta_ail_lef/1, Cl_delta_ail/1, Cl_elevator0/1, Cl/1, Cl_lef/1
  Cl_p/1 -> Subtract7/1
  beta (deg)/1 -> beta Prelookup/1, Product8/2
  Subtract2/1 -> Product1/1
  alpha Prelookup/2 -> Cl_r/2, dCl_r_lef/2, dCl_p_lef/2, dCl_beta/2, Cl_p/2, Cl_delta_r/2, Cl_delta_ail_lef/2, Cl_delta_ail/2, Cl/2, Cl_lef/2, Cl_elevator0/2
  alpha (deg)/1 -> alpha Prelookup/1
  Product/1 -> Subtract8/2
  Subtract6/1 -> Product5/2
  rb_2v/1 -> Product5/1
  Cl_delta_ail/1 -> Subtract1/1
  elevator Prelookup/1 -> Cl/5
  Product7/1 -> Subtract8/4
  Subtract7/1 -> Product7/1
  Product5/1 -> Subtract8/3
  dCl_r_lef/1 -> Product4/1
  Subtract3/1 -> Gain1/1
  dlef/1 -> Product6/1, Product4/2, Product/2, Product1/2
  Cl_delta_ail_lef/1 -> Subtract2/1
  beta Prelookup/2 -> Cl/4, Cl_lef/4, Cl_elevator0/4, Cl_delta_ail/4, Cl_delta_ail_lef/4, Cl_delta_r/4
  Product4/1 -> Subtract6/2
  dCl_beta/1 -> Product8/1
  Product1/1 -> Subtract5/2
  dCl_p_lef/1 -> Product6/2
  Product8/1 -> Subtract8/5
  Cl_r/1 -> Subtract6/1
  elevator Prelookup/2 -> Cl/6
  Cl/1 -> Subtract8/1
  pb_2v/1 -> Product7/2
  Subtract8/1 -> Cl_tot_hat/1
  Subtract5/1 -> Gain/1
  right elevator (deg)/1 -> Add/1
  left elevator (deg)/1 -> Add/2
  Add/1 -> Gain2/1
  Subtract1/1 -> [delta_Cl_delta_ail], Subtract2/3, Subtract5/1
  Gain1/1 -> Mux/5  "gp_dr1"
  [delta_Cl_delta_ail] -> Gain7/1
  Gain/1 -> Gain3/1
  Gain4/1 -> Mux/2  "gp_dla1"
  Mux/1 -> gr1/1, gp1/1
  Gain7/1 -> Gain8/1
  Gain8/1 -> Mux/3, Gain9/1  "gp_dre1"
  Gain9/1 -> Mux/4  "gp_dle1"
  Gain2/1 -> elevator Prelookup/1
  Gain3/1 -> Gain4/1, Mux/1  "gp_dla1"

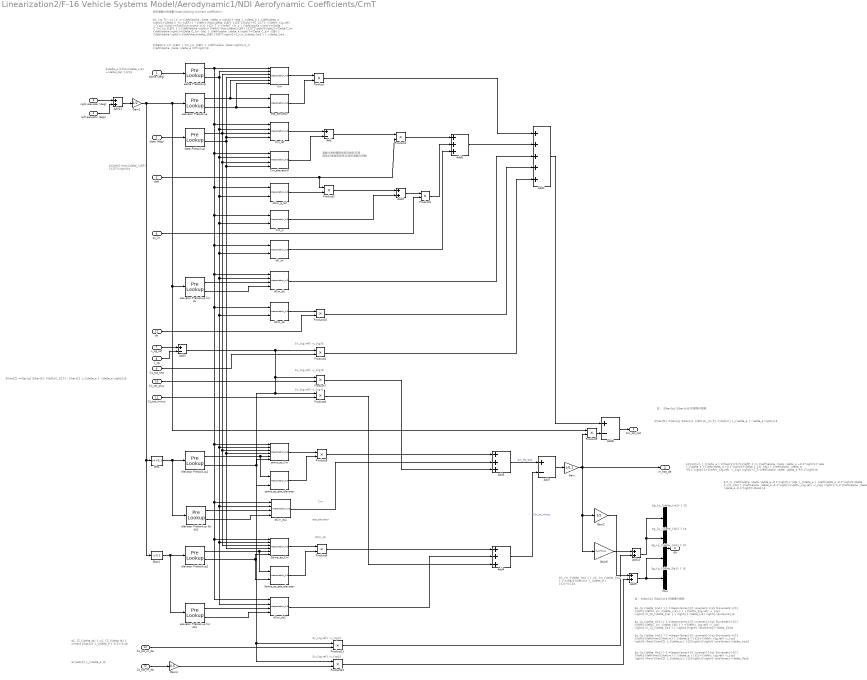
== system Linearization2/F-16 Vehicle Systems Model/Aerodynamic1/NDI Aerofynamic Coefficients/CmT ==
  note: $C_{m_{\delta_{ra} } } =C_{m_{\delta_{la} } } =\frac{{\hat{m} }_{\delta_e } }{2}∙0.12$
  note: $g_{q_{\delta_{ra1} } }$
  note: $g_{q_{\delta_{ra1} } } =\begin{array}{l} \overset{-}{q} S\overset{-}{C} {\left\{{\left(C_{m_{\delta_{ra} } } +{\left(x_{cg,ref} -x_{cg} \right)}∙C_{Z_{\delta_{ra} } } \right\}}∙\delta_{ra} \right)} \end{array}$
  note: $-C_m {\left(\alpha ,\beta ,\delta_e -0.1°\right)}{∙\eta }_{\delta_e } {\left(\delta_e -0.1°\right)}-\Delta C_{m_{ds} } {\left(\alpha ,\delta_e -0.1°\right)}-{\left(x_{cg,ref} -x_{cg} \right)}∙C_Z {\left(\alpha ,\beta ,\delta_e -0.1°\right)}\rbrack}$
  note: ${\hat{m} }_{\delta_e } =\frac{1}{0.2}{\left[\ C_m {\left(\alpha ,\beta ,\delta_e +0.1°\right)}{∙\eta }_{\delta_e } {\left(\delta_e +0.1°\right)}+\Delta C_{m_{ds} } {\left(\alpha ,\delta_e +0.1°\right)}}+{\left(x_{cg,ref} -x_{cg} \right)}∙C_Z {\left(\alpha ,\beta ,\delta_e +0.1°\right)}$
  note: $\hat{M} =\bar{q} S\bar{c} {\left\{C_{m,T} -{\hat{m} }_{\delta_e } ∙\delta_e \right\}}$
  note: dCm_ds
  note: $x_{cg,ref} -x_{cg}$
  note: eta_elevator
  note: Cm
  note: 氣動力表格僅提供到攻角到45度，
      | 超過45度後皆採用45度的氣動力係數
  note: $x_{cg,ref} -x_{cg}$
  note: $x_{cg,ref} -x_{cg}$
  note: $C_{m,T} \ =\ \ C_m {\left(\alpha ,\beta ,\delta_e \right)}{∙\eta }_{\delta_e } {\left(\delta_e \right)}+\Delta C_{m_{LEF} } ∙{\left(1-\frac{\delta_{LEF} }{25°}\right)}+C_{Z,T} ∙{\left(x_{cg,ref} -x_{cg} \right)}+\frac{q\overset{-}{c} }{2V_T }∙{\left[C_{m_q } {\left(\alpha \right)}+\Delta C_{m_{q_{LEF} } } {\left(\alpha \right)}∙{\left(1-\frac{\delta_{LEF} }{25°}\right)}\right]}+\Delta C_m {\left(\alpha \right)}+\Delta C_{m_{ds} } {\left(\alpha ,\delta_e \right)}+\Delta C_{m_{SB} } {\left(\alpha \right)}∙{\left(\frac{\delta_{SB} }{60°}\right)}+C_{m_{\delta_{ra} } } ∙\delta_{ra} +C_{m_{\delta_{la} } } ∙\delta_{la}$
  note: $\Delta C_{m_{LEF} } =C_{m_{LEF} } {\left(\alpha ,\beta \right)}-C_m {\left(\alpha ,\beta ,\delta_e =0°\right)}$
  note: 俯仰氣動力矩係數 (total pitching moment coefficient)：
  note: ${\left(1-\frac{\delta_{LEF} }{25°}\right)}$
  note: 註： $\bar{q} S\bar{c}$ 在模塊外面乘
  note: $\delta_e =\frac{\delta_{re} +\delta_{le} }{2}$
  note: $\hat{Z} =\bar{q} S\bar{C} {\left\{C_{Z,T} -{\hat{Z} }_{\delta_e } ∙\delta_e \right\}}$
  note: ${\hat{Z} }_{\delta_e }$
  note: $C_{Z_{\delta ra} } =C_{Z_{\delta la} } =\frac{{\hat{Z} }_{\delta_e } }{2}∙0.4$
  note: $g_{q_{\delta_{la1} } } =\begin{array}{l} \overset{-}{q} S\overset{-}{C} {\left\{{\left(C_{m_{\delta_{la} } } +{\left(x_{cg,ref} -x_{cg} \right)}∙C_{Z_{\delta_{la} } } \right\}}\right)} \end{array}∙\delta_{la}$
  note: $g_{q_{\delta_{re1} } } =\begin{array}{l} \overset{-}{q} S\overset{-}{C} {\left\{{\left(\frac{{\hat{m} }_{\delta_e } }{2}+{\left(x_{cg,ref} -x_{cg} \right)}∙\frac{{\hat{Z} }_{\delta_e } }{2}\right\}}\right)} \end{array}∙\delta_{re}$
  note: $g_{q_{\delta_{le1} } } =\begin{array}{l} \overset{-}{q} S\overset{-}{C} {\left\{{\left(\frac{{\hat{m} }_{\delta_e } }{2}+{\left(x_{cg,ref} -x_{cg} \right)}∙\frac{{\hat{Z} }_{\delta_e } }{2}\right\}}\right)} \end{array}∙\delta_{le}$
  note: 註： $\bar{q} S\bar{c}$ 在模塊外面乘
  note: $x_{cg,ref} -x_{cg}$
  note: $x_{cg,ref} -x_{cg}$
  note: $g_{q_{\delta_{la1} } }$
  note: $g_{q_{\delta_{re1} } }$
  note: $g_{q_{\delta_{le1} } }$
  alpha (deg) : Inport
  beta (deg) : Inport  Port=2
  right elevator (deg) : Inport  Port=3
  left elevator (deg) : Inport  Port=4
  dlef : Inport  Port=5
  qc_2v : Inport  Port=6
  x_cg_ref : Inport  Port=7
  x_cg : Inport  Port=8
  Cz_tot_hat : Inport  Port=9
  Cz_tot_plus : Inport  Port=10
  Cz_tot_minus : Inport  Port=11
  sb : Inport  Port=12
  Cz_tot_m_de : Inport  Port=13
  Cz_tot_m_da : Inport  Port=14
  Add{,3,7..8} (4 alike) : Sum  Inputs=+-
  Add1 : Sum  Inputs=+++++
  Add{2,9..11} (4 alike) : Sum
  Add4 : Sum  Inputs=+++
  Add5 : Sum  Inputs=+++
  Add6 : Sum  Inputs=+++
  Bias : Bias  Bias=+0.1  SaturateOnIntegerOverflow=off
  Bias1 : Bias  Bias=-0.1  SaturateOnIntegerOverflow=off
  Cm : Interpolation_n-D  NumberOfTableDimensions=3  Table=AeroCoeff.Cm
      settings: InputPortMap=u0,u1,u2,u3,u4,u5
  Cm_elevator0 : Interpolation_n-D  Table=AeroCoeff.Cm_elevator0
  Cm_lef : Interpolation_n-D  Table=AeroCoeff.Cm_lef
  Cm_q : Interpolation_n-D  NumberOfTableDimensions=1  Table=AeroCoeff.Cm_q
      settings: InputPortMap=u0,u1
  Gain : Gain  Gain=1/0.2
  Gain1 : Gain  Gain=1/2
  Gain2 : Gain  Gain=1/2
  Gain4 : Gain  Gain=0.5
  Gain6 : Gain  Gain=(1/2)*0.12
  Mux : Mux
  Product{,1..12} (13 alike) : Product
  Same_as_Cm : Interpolation_n-D  NumberOfTableDimensions=3  Table=AeroCoeff.Cm
      settings: InputPortMap=u0,u1,u2,u3,u4,u5
  Same_as_eta_elevator : Interpolation_n-D  NumberOfTableDimensions=1  Table=AeroCoeff.eta_elevator
      settings: InputPortMap=u0,u1
  alpha Prelookup : PreLookup  BreakpointsData=AeroCoeff.alpha_prelookup  IndexSearchMethod=Linear search  BeginIndexSearchUsingPreviousIndexResult=on  DiagnosticForOutOfRangeInput=Warning
  beta Prelookup : PreLookup  BreakpointsData=AeroCoeff.beta_prelookup  IndexSearchMethod=Linear search  BeginIndexSearchUsingPreviousIndexResult=on  DiagnosticForOutOfRangeInput=Warning
  dC_m : Interpolation_n-D  NumberOfTableDimensions=1  Table=AeroCoeff.dC_m
      settings: InputPortMap=u0,u1
  dCm_ds : Interpolation_n-D  Table=AeroCoeff.dCm_ds
  dCm_ds1 : Interpolation_n-D  Table=AeroCoeff.dCm_ds
  dCm_ds2 : Interpolation_n-D  Table=AeroCoeff.dCm_ds
  dCm_q_lef : Interpolation_n-D  NumberOfTableDimensions=1  Table=AeroCoeff.dCm_q_lef
      settings: InputPortMap=u0,u1
  dCm_sb : Interpolation_n-D  NumberOfTableDimensions=1  Table=AeroCoeff.dCm_sb
      settings: InputPortMap=u0,u1
  elevator Prelookup : PreLookup  BreakpointsData=AeroCoeff.elevator_prelookup2  IndexSearchMethod=Linear search  BeginIndexSearchUsingPreviousIndexResult=on  DiagnosticForOutOfRangeInput=Warning
  elevator Prelookup for ds : PreLookup  BreakpointsData=AeroCoeff.elevator_prelookup3  IndexSearchMethod=Linear search  BeginIndexSearchUsingPreviousIndexResult=on  DiagnosticForOutOfRangeInput=Warning
  elevator Prelookup for ds1 : PreLookup  BreakpointsData=AeroCoeff.elevator_prelookup3  IndexSearchMethod=Linear search  BeginIndexSearchUsingPreviousIndexResult=on  DiagnosticForOutOfRangeInput=Warning
  elevator Prelookup for ds2 : PreLookup  BreakpointsData=AeroCoeff.elevator_prelookup3  IndexSearchMethod=Linear search  BeginIndexSearchUsingPreviousIndexResult=on  DiagnosticForOutOfRangeInput=Warning
  elevator Prelookup1 : PreLookup  BreakpointsData=AeroCoeff.elevator_prelookup2  IndexSearchMethod=Linear search  BeginIndexSearchUsingPreviousIndexResult=on  DiagnosticForOutOfRangeInput=Warning
  elevator Prelookup2 : PreLookup  BreakpointsData=AeroCoeff.elevator_prelookup2  IndexSearchMethod=Linear search  BeginIndexSearchUsingPreviousIndexResult=on  DiagnosticForOutOfRangeInput=Warning
  eta_elevator : Interpolation_n-D  NumberOfTableDimensions=1  Table=AeroCoeff.eta_elevator
      settings: InputPortMap=u0,u1
  same_as_Cm : Interpolation_n-D  NumberOfTableDimensions=3  Table=AeroCoeff.Cm
      settings: InputPortMap=u0,u1,u2,u3,u4,u5
  same_as_eta_elevator : Interpolation_n-D  NumberOfTableDimensions=1  Table=AeroCoeff.eta_elevator
      settings: InputPortMap=u0,u1
  Cm_tot_hat : Outport  VectorParamsAs1DForOutWhenUnconnected=off
  m_hat_de : Outport  Port=2  VectorParamsAs1DForOutWhenUnconnected=off
  gq : Outport  Port=3  VectorParamsAs1DForOutWhenUnconnected=off
  wires:
  Cm/1 -> Product/1
  Cm_lef/1 -> Add/1
  Add3/1 -> Product12/1, Product11/1, Product8/1, Product7/1, Product4/1
  Product3/1 -> Add6/2
  Cm_elevator0/1 -> Add/2
  elevator Prelookup/1 -> Cm/5, eta_elevator/1
  dC_m/1 -> Add6/3
  dlef/1 -> Product2/1, Product1/2
  elevator Prelookup/2 -> Cm/6, eta_elevator/2
  right elevator (deg)/1 -> Add11/1
  Product1/1 -> Add6/1
  eta_elevator/1 -> Product/2
  beta Prelookup/2 -> Same_as_Cm/4, same_as_Cm/4, Cm_elevator0/4, Cm/4, Cm_lef/4
  Product2/1 -> Add2/1
  Cm_q/1 -> Add2/2
  beta Prelookup/1 -> Cm/3, Same_as_Cm/3, same_as_Cm/3, Cm_elevator0/3, Cm_lef/3
  Product/1 -> Add1/1
  dCm_q_lef/1 -> Product2/2
  Add2/1 -> Product3/1
  Add/1 -> Product1/1
  qc_2v/1 -> Product3/2
  alpha (deg)/1 -> alpha Prelookup/1
  Product4/1 -> Add1/5
  beta (deg)/1 -> beta Prelookup/1
  x_cg/1 -> Add3/2
  Add1/1 -> Add8/1
  Cz_tot_hat/1 -> Product4/2
  x_cg_ref/1 -> Add3/1
  Bias/1 -> elevator Prelookup for ds1/1, elevator Prelookup1/1
  Bias1/1 -> elevator Prelookup for ds2/1, elevator Prelookup2/1
  elevator Prelookup1/1 -> same_as_Cm/5, same_as_eta_elevator/1
  elevator Prelookup1/2 -> same_as_Cm/6, same_as_eta_elevator/2
  elevator Prelookup2/1 -> Same_as_eta_elevator/1, Same_as_Cm/5
  elevator Prelookup2/2 -> Same_as_Cm/6, Same_as_eta_elevator/2
  same_as_Cm/1 -> Product5/1
  same_as_eta_elevator/1 -> Product5/2
  Same_as_Cm/1 -> Product6/1
  Same_as_eta_elevator/1 -> Product6/2
  Product5/1 -> Add5/1
  Cz_tot_plus/1 -> Product7/2
  Cz_tot_minus/1 -> Product8/2
  Product7/1 -> Add5/3
  Product6/1 -> Add4/1
  Product8/1 -> Add4/3
  Add6/1 -> Add1/2
  Add5/1 -> Add7/1  "Cm_tot_plus"
  Add4/1 -> Add7/2  "Cm_tot_minus"
  Add7/1 -> Gain/1
  Product9/1 -> Add8/2
  Add8/1 -> Cm_tot_hat/1
  sb/1 -> Product10/2
  dCm_sb/1 -> Product10/1
  Product10/1 -> Add1/4
  elevator Prelookup for ds/1 -> dCm_ds/3
  elevator Prelookup for ds/2 -> dCm_ds/4
  dCm_ds/1 -> Add1/3
  elevator Prelookup for ds1/2 -> dCm_ds1/4
  elevator Prelookup for ds1/1 -> dCm_ds1/3
  alpha Prelookup/2 -> Cm/2, dCm_ds1/2, dCm_ds2/2, Same_as_Cm/2, same_as_Cm/2, dCm_sb/2, dCm_ds/2, dC_m/2, Cm_q/2, dCm_q_lef/2, Cm_elevator0/2, Cm_lef/2
  alpha Prelookup/1 -> dCm_ds1/1, dCm_ds2/1, Same_as_Cm/1, same_as_Cm/1, dCm_sb/1, dCm_ds/1, dC_m/1, Cm_q/1, dCm_q_lef/1, Cm_elevator0/1, Cm_lef/1, Cm/1
  elevator Prelookup for ds2/1 -> dCm_ds2/3
  elevator Prelookup for ds2/2 -> dCm_ds2/4
  dCm_ds1/1 -> Add5/2
  dCm_ds2/1 -> Add4/2
  Gain/1 -> m_hat_de/1, Gain2/1, Gain6/1, Product9/2
  Mux/1 -> gq/1
  Cz_tot_m_da/1 -> Product11/2
  Cz_tot_m_de/1 -> Gain4/1
  Gain2/1 -> Add9/1
  Product12/1 -> Add9/2
  Add9/1 -> Mux/4, Mux/3
  Gain6/1 -> Add10/1
  Product11/1 -> Add10/2
  Add10/1 -> Mux/1, Mux/2
  left elevator (deg)/1 -> Add11/2
  Add11/1 -> Gain1/1
  Gain1/1 -> Bias1/1, Bias/1, elevator Prelookup/1, elevator Prelookup for ds/1, Product9/1
  Gain4/1 -> Product12/2
